simulink model "Buck_converter_step3"  (Simulink 8.4)
settings: Solver=ode23tb  StartTime=0.0  StopTime=0.01  MaxStep=1e-6  RelTol=1e-4
PreLoadFcn:
  | Ts = 2e-6
  | Tsc = 1e-7
libraries: powerlib x12
settings Model: Creator=kfukui  LastModifiedBy=kotsuka
settings OptimizationCC: BlockReduction=off  ConditionallyExecuteInputs=off
settings DebuggingCC: SingleTaskRateTransMsg=error  ParameterUnderflowMsg=warning  FcnCallInpInsideContextMsg=EnableAllAsWarning

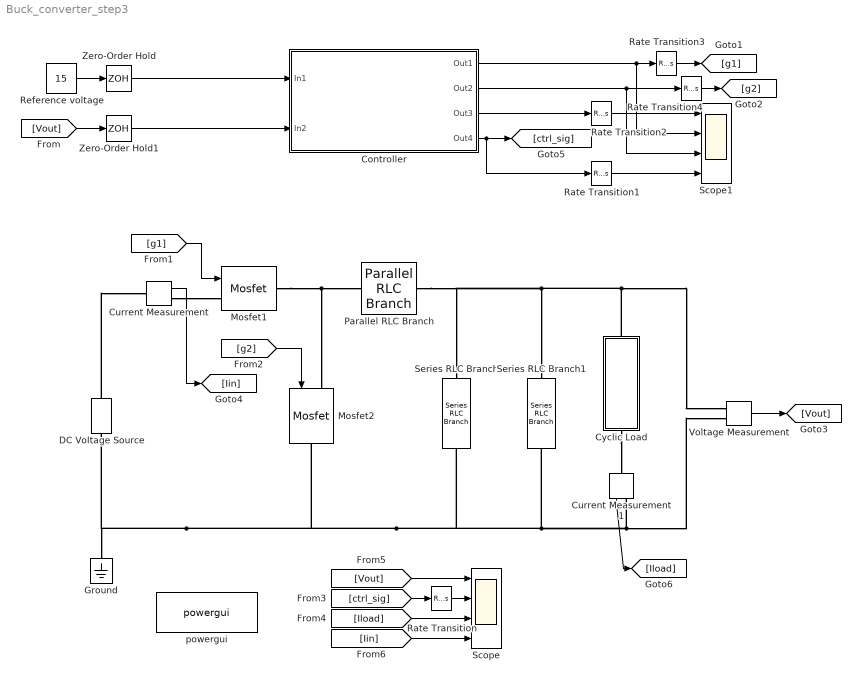
== system Buck_converter_step3 ==
  Controller : Subsystem
  Current Measurement : powerlib/Measurements/Current Measurement  PhasorSimulation=off  OutputType=Complex  PSBequivalent=0
  Current Measurement1 : powerlib/Measurements/Current Measurement  PhasorSimulation=off  OutputType=Complex  PSBequivalent=0
  Cyclic Load : Subsystem
  DC Voltage Source : powerlib/Electrical Sources/DC Voltage Source  Amplitude=30  Measurements=None
  Ground : powerlib/Elements/Ground  LConnTagsString=a
  Mosfet1 : powerlib/Power Electronics/Mosfet  Ron=0.1  Lon=0  Rd=0.01  Vfd=0.8  IC=0  Rs=1e5  Cs=inf  Measurements=off
  Mosfet2 : powerlib/Power Electronics/Mosfet  Ron=0.1  Lon=0  Rd=0.01  Vfd=0.8  IC=0  Rs=1e5  Cs=inf  Measurements=off
  Parallel RLC Branch : powerlib/Elements/Parallel RLC Branch  LConnTagsString=a  RConnTagsString=__new0  BranchType=RL  Resistance=10e3  Inductance=1e-3  SetiL0=off  InitialCurrent=0  Capacitance=1e-6  Setx0=off  InitialVoltage=0  Measurements=None
  Rate Transition{,1..4} (5 alike) : RateTransition  Deterministic=off
  Reference voltage : Constant  Value=15
  Scope : Scope  NumInputPorts=4
      settings: TimeRange=0.01  YMin=0~0~0~0  YMax=20~1~2~8
  Scope1 : Scope  NumInputPorts=4
      settings: TimeRange=0.01  YMin=-1~0~0~0  YMax=1~1~1~1
  Series RLC Branch : powerlib/Elements/Series RLC Branch  LConnTagsString=__new0  RConnTagsString=__new0  BranchType=C  Resistance=1  Inductance=1e-3  SetiL0=off  InitialCurrent=0  Capacitance=22e-6  Setx0=off  InitialVoltage=0  Measurements=None
  Series RLC Branch1 : powerlib/Elements/Series RLC Branch  LConnTagsString=__new0  RConnTagsString=__new0  BranchType=R  Resistance=3.75  Inductance=1e-3  SetiL0=off  InitialCurrent=0  Capacitance=22e-6  Setx0=off  InitialVoltage=0  Measurements=None
  Voltage Measurement : powerlib/Measurements/Voltage Measurement  PhasorSimulation=off  OutputType=Complex  PSBequivalent=0
  Zero-Order Hold : ZeroOrderHold  SampleTime=Ts
  Zero-Order Hold1 : ZeroOrderHold  SampleTime=Ts
  powergui : powerlib/powergui  Priority=1  SimulationMode=Continuous  SolverType=Tustin  SampleTime=50e-6  frequency=60  SPID=off  DisableSnubberDevices=off  DisableRonSwitches=off  DisableVfSwitches=off  SwTol=0  DisplayEquations=off  Interpol=off  methode=off  Ts=100  frequencyindice=0  Pbase=100e6  ErrMax=1e-4  Iterations=50  UnitsV=kV  UnitsW=MW  FunctionMessages=off  echomessages=off  HookPort=off  EnableUseOfTLC=off  x0status=blocks  RestoreLinks=warning  ResistiveCurrentMeasurement=off  Frange=[0:2:500]  Ylog=off  Xlog=on  ShowGrid=off  save=off  variable=ZData  structure=0  ZoomFFT=off  StartTime=0.0  cycles=1  DisplayStyle=1  fundamental=60  FreqAxis=off  MaxFrequency=1000  frequencyindicesteady=1  RmsSteady=1  display=off
  wires:
  Voltage Measurement/1 -> [Vout]
  Reference voltage/1 -> Zero-Order Hold/1
  [Vout] -> Zero-Order Hold1/1
  Controller/1(Out1) -> Scope1/2, Rate Transition3/1
  Controller/2(Out2) -> Scope1/3, Rate Transition4/1
  [g1] -> Mosfet1/1
  [g2] -> Mosfet2/1
  Current Measurement/1 -> [Iin]
  Current Measurement1/1 -> [Iload]
  [Vout] -> Scope/1
  [ctrl_sig] -> Rate Transition/1
  [Iload] -> Scope/3
  [Iin] -> Scope/4
  Controller/3(Out3) -> Rate Transition2/1
  Controller/4(Out4) -> [ctrl_sig], Rate Transition1/1
  Rate Transition/1 -> Scope/2
  Rate Transition1/1 -> Scope1/4
  Rate Transition2/1 -> Scope1/1
  Rate Transition3/1 -> [g1]
  Rate Transition4/1 -> [g2]
  Zero-Order Hold/1 -> Controller/1(In1)
  Zero-Order Hold1/1 -> Controller/2(In2)
  connections:
  DC Voltage Source/RConn1 -- Current Measurement/LConn1
  Current Measurement/RConn1 -- Mosfet1/LConn1
  Mosfet1/RConn1 -- Mosfet2/LConn1 -- Parallel RLC Branch/LConn1
  Cyclic Load/LConn1 -- Parallel RLC Branch/RConn1 -- Series RLC Branch/LConn1 -- Series RLC Branch1/LConn1 -- Voltage Measurement/LConn1
  Series RLC Branch1/RConn1 -- Series RLC Branch/RConn1 -- Mosfet2/RConn1 -- DC Voltage Source/LConn1 -- Ground/LConn1 -- Current Measurement1/RConn1 -- Voltage Measurement/LConn2
  Cyclic Load/RConn1 -- Current Measurement1/LConn1

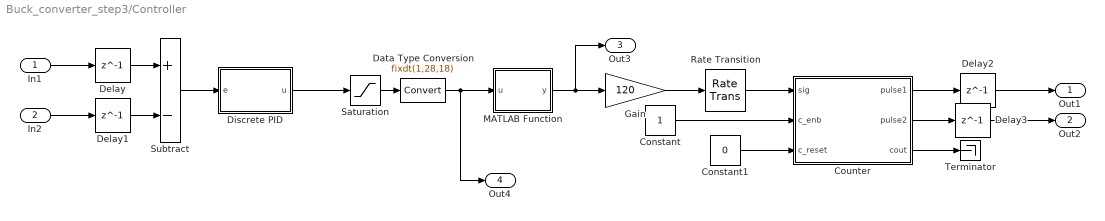
== system Buck_converter_step3/Controller ==
  In1 : Inport
  In2 : Inport  Port=2
  Constant : Constant  OutDataTypeStr=boolean  SampleTime=Tsc
  Constant1 : Constant  Value=0  OutDataTypeStr=boolean  SampleTime=Tsc
  Counter : MATLAB Function  TreatAsAtomicUnit=on
  Data Type Conversion : DataTypeConversion  OutDataTypeStr=fixdt(1,28,18)
  Delay{,1..3} (4 alike) : Delay  DelayLength=1
  Discrete PID : Subsystem
  Gain : Gain  Gain=120  OutDataTypeStr=fixdt(1,24,15)  RndMeth=Nearest
  MATLAB Function : MATLAB Function  TreatAsAtomicUnit=on
  Rate Transition : RateTransition  OutPortSampleTime=Tsc
  Saturation : Saturate  UpperLimit=0.95  LowerLimit=0.01  OutDataTypeStr=Inherit: Inherit via back propagation
  Subtract : Sum  Inputs=+-  RndMeth=Nearest  OutDataTypeStr=Inherit: Same as first input
  Terminator : Terminator
  Out1 : Outport
  Out2 : Outport  Port=2
  Out3 : Outport  Port=3
  Out4 : Outport  Port=4
  wires:
  MATLAB Function/1(y) -> Out3/1, Gain/1
  Saturation/1 -> Data Type Conversion/1
  Discrete PID/1(u) -> Saturation/1
  Subtract/1 -> Discrete PID/1(e)
  In1/1 -> Delay/1
  In2/1 -> Delay1/1
  Counter/1(pulse1) -> Delay2/1
  Counter/2(pulse2) -> Delay3/1
  Constant/1 -> Counter/2(c_enb)
  Constant1/1 -> Counter/3(c_reset)
  Rate Transition/1 -> Counter/1(sig)
  Gain/1 -> Rate Transition/1
  Counter/3(cout) -> Terminator/1
  Delay/1 -> Subtract/1
  Delay1/1 -> Subtract/2
  Delay2/1 -> Out1/1
  Delay3/1 -> Out2/1
  Data Type Conversion/1 -> MATLAB Function/1(u), Out4/1

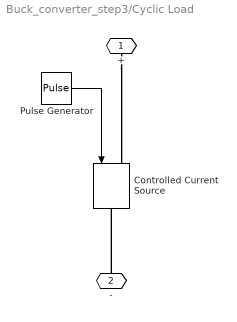
== system Buck_converter_step3/Cyclic Load ==
  Controlled Current Source : powerlib/Electrical Sources/Controlled Current Source  Initialize=on  Source_Type=AC  Amplitude=0  Phase=0  Frequency=0  Measurements=None
  Pulse Generator : DiscretePulseGenerator  PulseType=Time based  Amplitude=2  Period=1/200  PulseWidth=50  PhaseDelay=1/400
  + : PMIOPort  Port=1  Side=Left
  - : PMIOPort  Port=2  Side=Right
  wires:
  Pulse Generator/1 -> Controlled Current Source/1
  connections:
  +/RConn1 -- Controlled Current Source/LConn1
  -/RConn1 -- Controlled Current Source/RConn1

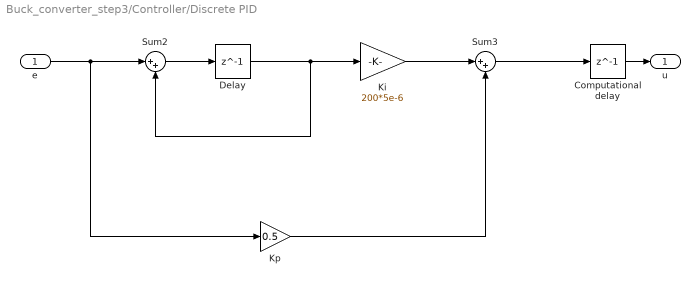
== system Buck_converter_step3/Controller/Discrete PID ==
  e : Inport
  Computational delay : Delay  DelayLength=1  InputProcessing=Inherited
  Delay : Delay  DelayLength=1  InputProcessing=Inherited
  Ki : Gain  Gain=200*5e-6  OutDataTypeStr=Inherit: Same as input
  Kp : Gain  Gain=0.5  OutDataTypeStr=Inherit: Same as input
  Sum2 : Sum  Inputs=|++  SaturateOnIntegerOverflow=on
  Sum3 : Sum  Inputs=|++  SaturateOnIntegerOverflow=on  OutDataTypeStr=Inherit: Same as first input
  u : Outport
  wires:
  Computational delay/1 -> u/1
  Ki/1 -> Sum3/1
  Kp/1 -> Sum3/2
  Sum3/1 -> Computational delay/1
  Delay/1 -> Sum2/2, Ki/1
  Sum2/1 -> Delay/1
  e/1 -> Kp/1, Sum2/1

== matlab function Controller/Counter ==
  data: sig input double; pulse1 output boolean; c_enb input double; c_reset input double; pulse2 output boolean; cout output int8
function [pulse1,pulse2, cout] = fcn(sig, c_enb, c_reset)
%#codegen

coutmax = int8(124);
dtime = 4; % samples
persistent ctmp;
if isempty(ctmp)
	ctmp = int8(0);
	dtime_count = fi(0,0,4);
end
if c_reset
	ctmp = int8(0);
else
	if c_enb
		if ctmp < coutmax
			ctmp = int8(ctmp+1);
		else
			ctmp = int8(-125);
		end
	end
end
cout = ctmp;

if ctmp < sig
	pulse1 = true;
	pulse2 = false;
else
	pulse1 = false;
	pulse2 = true;
end

== matlab function Controller/MATLAB Function ==
  data: u input double; y output double
function y = fcn(u)
%#codegen

fisetting = numerictype(u);
tmp = fi(2*u,fisetting);
y = fi(tmp-1,fisetting);
